simulink model "simulation_w_switch_sln3"  (Simulink 10.1)
settings: Solver=VariableStepAuto  StartTime=0.0  StopTime=tTot  MaxStep=1e-5  RelTol=1e-5
PreLoadFcn:
  | syst_init
values from neighbouring files (symbols this model uses):
  Aij = Aconn-Aii    [syst_init.m]
  AL = blkdiag(DGU.ALi)    [syst_init.m]
  atk24 = [zeros(3,1); 0.1*rand(3,1)-0.05]    [syst_init.m]
  atk34 = [zeros(3,1); 0.1*rand(3,1)-0.05]    [syst_init.m]
  B = blkdiag(DGU.B)    [syst_init.m]
  bC = blkdiag(DGU.bC)    [syst_init.m]
  bF = blkdiag(DGU.bF)    [syst_init.m]
  bH = blkdiag(DGU.bH)    [syst_init.m]
  bigCyComm = [zeros(3,3)  eye(3) zeros(3,30) ... (first row only)    [syst_init.m]
  bKhat = blkdiag(DGU.bKhat)    [syst_init.m]
  DGU = stateDyn(DGU,6)    [syst_init.m]
  F = blkdiag(DGU.Fj)    [syst_init.m]
  H = blkdiag(DGU.Hj)    [syst_init.m]
  K = blkdiag(DGU.K)    [syst_init.m]
  Khat = blkdiag(DGU.Khat)    [syst_init.m]
  L = blkdiag(DGU.Li)    [syst_init.m]
  n = 3    [syst_init.m]
  N = 6    [syst_init.m]
  nMaxMeas = .01    (= 0.01)    [syst_init.m]
  rhoMax = nMaxMeas*repmat([ones(n-1,1);0],N,1)    [syst_init.m]
  T = blkdiag(DGU.Tj)    [syst_init.m]
  Ta = 8    [syst_init.m]
  Tc = 2    [syst_init.m]
  tSampData = 1e-3    (= 0.001)    [syst_init.m]
  Vs = 60    [syst_init.m]
  wMax = nMax*repmat([ones(n-1,1);0],N,1)+nMaxMeas*repmat([zeros(n-1,1);1],N,1)    [syst_init.m]
undefined symbols (not defined in the file or in its folder): epsilon0bar, integral_Loc, rLoc_bar
libraries: powerlib x136, powerlib_meascontrol x13
(part 2 of 4)

== system simulation_w_switch_sln3/DGU5 ==
  note: Noisy Measurements
  note: State Computation
  note: Average Dynamics
  AC Current Source : powerlib/Electrical Sources/AC Current Source  Amplitude=18  Phase=90  Frequency=0  SampleTime=0  Measurements=Current
      settings: SourceProductBaseCode=PS
  Attack Detection Logic : Subsystem
  Capacitance : powerlib/Elements/Series RLC Branch  LConnTagsString=__new0  RConnTagsString=__new0  BranchType=C  Resistance=1  Inductance=1.8e-3  SetiL0=off  InitialCurrent=0  Capacitance=DGU(5).Ct  Setx0=off  InitialVoltage=48  Measurements=Branch voltage and current
  Current Measurement : powerlib/Measurements/Current Measurement  PhasorSimulation=off  OutputType=Magnitude  PSBequivalent=0
  DC Voltage Source : powerlib/Electrical Sources/DC Voltage Source  Amplitude=Vs  Measurements=Voltage
  Diode : powerlib/Power Electronics/Diode  Ron=0.001  Lon=0  Vf=0.8  IC=0  UseSnubber=0  Rs=500  Cs=250e-9  Measurements=off
  Diode1 : powerlib/Power Electronics/Diode  Ron=0.001  Lon=0  Vf=0.8  IC=0  UseSnubber=0  Rs=500  Cs=250e-9  Measurements=off
  Gain1 : Gain  Gain=[1 0 0]  Multiplication=Matrix(K*u) (u vector)
  Gain4 : Gain  Gain=[zeros(3,n*4) eye(3) zeros(3,n*1)]  Multiplication=Matrix(K*u) (u vector)
  Ground : powerlib/Elements/Ground  LConnTagsString=a
  Ground1 : powerlib/Elements/Ground  LConnTagsString=a
  IGBT : powerlib/Power Electronics/IGBT  Ron=0.001  Lon=0  Vf=1  Tf=1e-6  Tt=2e-6  IC=0  Rs=1e5  Cs=inf  Measurements=on
  IGBT1 : powerlib/Power Electronics/IGBT  Ron=0.001  Lon=0  Vf=1  Tf=1e-6  Tt=2e-6  IC=0  Rs=1e5  Cs=inf  Measurements=on
  Inductance : powerlib/Elements/Series RLC Branch  LConnTagsString=__new0  RConnTagsString=__new0  BranchType=L  Resistance=1  Inductance=DGU(5).Lt  SetiL0=off  InitialCurrent=18  Capacitance=1e-6  Setx0=off  InitialVoltage=0  Measurements=None
  Integrator : Integrator
  Luenberger  Observer : Subsystem
  Multimeter : powerlib/Measurements/Multimeter  PhasorSimulation=off  OutputType=Complex  sel=11  L=30  Gain=1  yselected={'Usrc: DGU5/DC Voltage Source'};  PSBOutputType=1  PSBequivalent=0  AxesSetting=[0,0.1,-100,100]  Display=0  SavedBlockNames=-11
  Multimeter1 : powerlib/Measurements/Multimeter  PhasorSimulation=off  OutputType=Complex  sel=18  L=30  Gain=1  yselected={'Ib: DGU5/Resistance'};  PSBOutputType=1  PSBequivalent=0  AxesSetting=[0,0.1,-100,100]  Display=0  SavedBlockNames=-11
  Multimeter2 : powerlib/Measurements/Multimeter  PhasorSimulation=off  OutputType=Complex  sel=17  L=30  Gain=1  yselected={'Ib: DGU5/Capacitance'};  PSBOutputType=1  PSBequivalent=0  AxesSetting=[0,0.1,-100,100]  Display=0  SavedBlockNames=-11
  Multimeter3 : powerlib/Measurements/Multimeter  PhasorSimulation=off  OutputType=Complex  sel=29  L=30  Gain=1  yselected={'Isrc: DGU5/AC Current Source'};  PSBOutputType=1  PSBequivalent=0  AxesSetting=[0,0.1,-100,100]  Display=0  SavedBlockNames=-11
  Multimeter5 : powerlib/Measurements/Multimeter  PhasorSimulation=off  OutputType=Complex  sel=3  L=30  Gain=1  yselected={'Ub: DGU5/Capacitance'};  PSBOutputType=1  PSBequivalent=0  AxesSetting=[0,0.1,-100,100]  Display=0  SavedBlockNames=-11
  Mux1 : Mux
  Mux4 : Mux  Inputs=3
  Primary  Voltage  Controller : Subsystem
  Product : Product  Multiplication=Matrix(*)
  Resistance : powerlib/Elements/Series RLC Branch  LConnTagsString=__new0  RConnTagsString=__new0  BranchType=R  Resistance=DGU(5).Rt  Inductance=1e-3  SetiL0=off  InitialCurrent=0  Capacitance=1e-6  Setx0=off  InitialVoltage=0  Measurements=Branch current
  Scope{,1..4,7} (6 alike) : Scope
  Secondary Consensus Layer : Subsystem
  State-Space1 : StateSpace  A=DGU(5).Aii  B=[DGU(5).M DGU(5).B [-1/DGU(5).Ct;0;0]]  C=eye(3)  D=zeros(n,4)  InitialCondition=0
  Sum2 : Sum  Inputs=|++
  Sum3 : Sum  Inputs=|+-
  Switching : Subsystem
  To Workspace : ToWorkspace  Commented=on  VariableName=x5  SaveFormat=Timeseries  SampleTime=tSampData
  To Workspace1 : ToWorkspace  Commented=on  VariableName=y5  SaveFormat=Timeseries  SampleTime=tSampData
  UIO : Subsystem
  Voltage Measurement : powerlib/Measurements/Voltage Measurement  PhasorSimulation=off  OutputType=Complex  PSBequivalent=0
  powergui1 : powerlib/powergui  Priority=1  Commented=on  SimulationMode=Continuous  SampleTime=50e-6  frequency=60  Iterations=50  frequencyindice=60  Pbase=100e6  ErrMax=1e-4  UnitsV=kV  UnitsW=MW  buscounter=0  FunctionMessages=off  echomessages=off  EnableUseOfTLC=off  CurrentSourceSwitches=off  DisableSnubberDevices=off  DisableRonSwitches=off  DisableVfSwitches=off  DisplayEquations=off  AutomaticDiscreteSolvers=off  SolverType=Tustin/Backward Euler (TBE)  Interpol=off  ExternalGateDelay=off  methode=off  Ts=100  x0status=blocks  SPID=on  SwTol=0  HookPort=off  NonlinearTolerance=1e-4  nMaxIteration=100  ContinueOnMaxIteration=off  RestoreLinks=warning  ResistiveCurrentMeasurement=off  Frange=[0:2:500]  Ylog=off  Xlog=on  ShowGrid=off  save=off  variable=ZData  structure=0  ZoomFFT=off  StartTime=0.0  cycles=1  DisplayStyle=1  fundamental=60  FreqAxis=off  MaxFrequency=1000  frequencyindicesteady=1  RmsSteady=1  display=off
  PCC5 : PMIOPort  Tag=PMCPort  Side=Left
  tag scope: Ic5=global, Il5=global, Inet5=global, It5=global, V5=global, Vs5=global, Vt5=global, x5=global, xavg5=global, y5=global
  wires:
  Multimeter/1 -> Scope/1, [Vs5]
  Multimeter2/1 -> Scope2/1, [Ic5]
  Voltage Measurement/1 -> Scope4/1, [Vt5]
  Multimeter1/1 -> Scope1/1, [It5]
  [SW_Buck_5n] -> IGBT1/1
  Multimeter3/1 -> Scope3/1, [Il5]
  [SW_Buck_5] -> IGBT/1
  Multimeter5/1 -> [V5]
  [x5] -> Sum2/2
  Sum3/1 -> Integrator/1
  Mux4/1 -> To Workspace/1, [x5]
  Sum2/1 -> To Workspace1/1, [y5]
  Integrator/1 -> Mux4/3
  Gain1/1 -> Sum3/2
  [It5] -> Mux4/2
  Gain4/1 -> Sum2/1, Scope7/1
  [y5] -> Gain1/1
  [Vref5] -> Sum3/1
  [rho] -> Gain4/1
  [V5] -> Mux4/1
  [Il5] -> Mux1/1
  Mux1/1 -> State-Space1/1
  [secondary] -> Product/2
  Current Measurement/1 -> [Inet5]
  Product/1 -> Mux1/4
  [Inet5] -> Product/1
  [Vref5] -> Mux1/2
  [Vt5d] -> Mux1/3
  State-Space1/1 -> [xavg5]
  connections:
  Ground1/LConn1 -- Voltage Measurement/LConn2
  IGBT1/RConn1 -- AC Current Source/RConn1 -- Capacitance/RConn1 -- Ground/LConn1 -- DC Voltage Source/LConn1 -- Diode1/LConn1
  Capacitance/LConn1 -- Current Measurement/LConn1 -- AC Current Source/LConn1 -- Inductance/RConn1
  IGBT/LConn1 -- Diode/RConn1 -- DC Voltage Source/RConn1
  Resistance/RConn1 -- Inductance/LConn1
  IGBT/RConn1 -- Resistance/LConn1 -- Voltage Measurement/LConn1 -- Diode1/RConn1 -- IGBT1/LConn1 -- Diode/LConn1
  PCC5/RConn1 -- Current Measurement/RConn1

== system simulation_w_switch_sln3/DGU6 ==
  note: Noisy Measurements
  note: State Computation
  note: Average Dynamics
  AC Current Source : powerlib/Electrical Sources/AC Current Source  Amplitude=16  Phase=90  Frequency=0  SampleTime=0  Measurements=Current
      settings: SourceProductBaseCode=PS
  Attack Detection Logic : Subsystem
  Capacitance : powerlib/Elements/Series RLC Branch  LConnTagsString=__new0  RConnTagsString=__new0  BranchType=C  Resistance=1  Inductance=1.8e-3  SetiL0=off  InitialCurrent=0  Capacitance=DGU(6).Ct  Setx0=off  InitialVoltage=48  Measurements=Branch voltage and current
  Current Measurement : powerlib/Measurements/Current Measurement  PhasorSimulation=off  OutputType=Magnitude  PSBequivalent=0
  DC Voltage Source : powerlib/Electrical Sources/DC Voltage Source  Amplitude=Vs  Measurements=Voltage
  Diode : powerlib/Power Electronics/Diode  Ron=0.001  Lon=0  Vf=0.8  IC=0  UseSnubber=0  Rs=500  Cs=250e-9  Measurements=off
  Diode1 : powerlib/Power Electronics/Diode  Ron=0.001  Lon=0  Vf=0.8  IC=0  UseSnubber=0  Rs=500  Cs=250e-9  Measurements=off
  Gain1 : Gain  Gain=[1 0 0]  Multiplication=Matrix(K*u) (u vector)
  Gain4 : Gain  Gain=[zeros(3,n*5) eye(3)]  Multiplication=Matrix(K*u) (u vector)
  Ground : powerlib/Elements/Ground  LConnTagsString=a
  Ground1 : powerlib/Elements/Ground  LConnTagsString=a
  IGBT : powerlib/Power Electronics/IGBT  Ron=0.001  Lon=0  Vf=1  Tf=1e-6  Tt=2e-6  IC=0  Rs=1e5  Cs=inf  Measurements=on
  IGBT1 : powerlib/Power Electronics/IGBT  Ron=0.001  Lon=0  Vf=1  Tf=1e-6  Tt=2e-6  IC=0  Rs=1e5  Cs=inf  Measurements=on
  Inductance : powerlib/Elements/Series RLC Branch  LConnTagsString=__new0  RConnTagsString=__new0  BranchType=L  Resistance=1  Inductance=DGU(6).Lt  SetiL0=off  InitialCurrent=16  Capacitance=1e-6  Setx0=off  InitialVoltage=0  Measurements=None
  Integrator : Integrator
  Luenberger  Observer1 : Subsystem
  Multimeter : powerlib/Measurements/Multimeter  PhasorSimulation=off  OutputType=Complex  sel=12  L=30  Gain=1  yselected={'Usrc: DGU6/DC Voltage Source'};  PSBOutputType=1  PSBequivalent=0  AxesSetting=[0,0.1,-100,100]  Display=0  SavedBlockNames=-11
  Multimeter1 : powerlib/Measurements/Multimeter  PhasorSimulation=off  OutputType=Complex  sel=20  L=30  Gain=1  yselected={'Ib: DGU6/Resistance'};  PSBOutputType=1  PSBequivalent=0  AxesSetting=[0,0.1,-100,100]  Display=0  SavedBlockNames=-11
  Multimeter2 : powerlib/Measurements/Multimeter  PhasorSimulation=off  OutputType=Complex  sel=19  L=30  Gain=1  yselected={'Ib: DGU6/Capacitance'};  PSBOutputType=1  PSBequivalent=0  AxesSetting=[0,0.1,-100,100]  Display=0  SavedBlockNames=-11
  Multimeter3 : powerlib/Measurements/Multimeter  PhasorSimulation=off  OutputType=Complex  sel=30  L=30  Gain=1  yselected={'Isrc: DGU6/AC Current Source'};  PSBOutputType=1  PSBequivalent=0  AxesSetting=[0,0.1,-100,100]  Display=0  SavedBlockNames=-11
  Multimeter6 : powerlib/Measurements/Multimeter  PhasorSimulation=off  OutputType=Complex  sel=4  L=30  Gain=1  yselected={'Ub: DGU6/Capacitance'};  PSBOutputType=1  PSBequivalent=0  AxesSetting=[0,0.1,-100,100]  Display=0  SavedBlockNames=-11
  Mux1 : Mux
  Mux4 : Mux  Inputs=3
  Primary  Voltage  Controller : Subsystem
  Product : Product  Multiplication=Matrix(*)
  Resistance : powerlib/Elements/Series RLC Branch  LConnTagsString=__new0  RConnTagsString=__new0  BranchType=R  Resistance=DGU(6).Rt  Inductance=1e-3  SetiL0=off  InitialCurrent=0  Capacitance=1e-6  Setx0=off  InitialVoltage=0  Measurements=Branch current
  Scope{,1..4,7} (6 alike) : Scope
  Secondary Consensus Layer : Subsystem
  State-Space1 : StateSpace  A=DGU(6).Aii  B=[DGU(6).M DGU(6).B [-1/DGU(6).Ct;0;0]]  C=eye(3)  D=zeros(n,4)  InitialCondition=0
  Sum2 : Sum  Inputs=|++
  Sum3 : Sum  Inputs=|+-
  Switching : Subsystem
  To Workspace : ToWorkspace  Commented=on  VariableName=x6  SaveFormat=Timeseries  SampleTime=tSampData
  To Workspace1 : ToWorkspace  Commented=on  VariableName=y6  SaveFormat=Timeseries  SampleTime=tSampData
  UIO1 : Subsystem
  Voltage Measurement : powerlib/Measurements/Voltage Measurement  PhasorSimulation=off  OutputType=Complex  PSBequivalent=0
  powergui1 : powerlib/powergui  Priority=1  Commented=on  SimulationMode=Continuous  SampleTime=50e-6  frequency=60  Iterations=50  frequencyindice=60  Pbase=100e6  ErrMax=1e-4  UnitsV=kV  UnitsW=MW  buscounter=0  FunctionMessages=off  echomessages=off  EnableUseOfTLC=off  CurrentSourceSwitches=off  DisableSnubberDevices=off  DisableRonSwitches=off  DisableVfSwitches=off  DisplayEquations=off  AutomaticDiscreteSolvers=off  SolverType=Tustin/Backward Euler (TBE)  Interpol=off  ExternalGateDelay=off  methode=off  Ts=100  x0status=blocks  SPID=on  SwTol=0  HookPort=off  NonlinearTolerance=1e-4  nMaxIteration=100  ContinueOnMaxIteration=off  RestoreLinks=warning  ResistiveCurrentMeasurement=off  Frange=[0:2:500]  Ylog=off  Xlog=on  ShowGrid=off  save=off  variable=ZData  structure=0  ZoomFFT=off  StartTime=0.0  cycles=1  DisplayStyle=1  fundamental=60  FreqAxis=off  MaxFrequency=1000  frequencyindicesteady=1  RmsSteady=1  display=off
  PCC6 : PMIOPort  Tag=PMCPort  Side=Right
  tag scope: Ic6=global, Il6=global, Inet6=global, It6=global, V6=global, Vs6=global, Vt6=global, x6=global, xavg6=global, y6=global
  wires:
  Multimeter/1 -> Scope/1, [Vs6]
  Multimeter2/1 -> Scope2/1, [Ic6]
  Voltage Measurement/1 -> Scope4/1, [Vt6]
  Multimeter1/1 -> Scope1/1, [It6]
  [SW_Buck_6n] -> IGBT1/1
  Multimeter3/1 -> Scope3/1, [Il6]
  [SW_Buck_6] -> IGBT/1
  Multimeter6/1 -> [V6]
  [x6] -> Sum2/2
  Sum3/1 -> Integrator/1
  Mux4/1 -> To Workspace/1, [x6]
  Sum2/1 -> To Workspace1/1, [y6]
  Integrator/1 -> Mux4/3
  Gain1/1 -> Sum3/2
  [It6] -> Mux4/2
  Gain4/1 -> Sum2/1, Scope7/1
  [y6] -> Gain1/1
  [Vref6] -> Sum3/1
  [rho] -> Gain4/1
  [V6] -> Mux4/1
  [Il6] -> Mux1/1
  Mux1/1 -> State-Space1/1
  [secondary] -> Product/2
  Current Measurement/1 -> [Inet6]
  Product/1 -> Mux1/4
  [Inet6] -> Product/1
  [Vref6] -> Mux1/2
  [Vt6d] -> Mux1/3
  State-Space1/1 -> [xavg6]
  connections:
  Ground1/LConn1 -- Voltage Measurement/LConn2
  IGBT1/RConn1 -- AC Current Source/RConn1 -- Capacitance/RConn1 -- Ground/LConn1 -- DC Voltage Source/LConn1 -- Diode1/LConn1
  Capacitance/LConn1 -- Current Measurement/LConn1 -- AC Current Source/LConn1 -- Inductance/RConn1
  IGBT/LConn1 -- Diode/RConn1 -- DC Voltage Source/RConn1
  Resistance/RConn1 -- Inductance/LConn1
  IGBT/RConn1 -- Resistance/LConn1 -- Voltage Measurement/LConn1 -- Diode1/RConn1 -- IGBT1/LConn1 -- Diode/LConn1
  PCC6/RConn1 -- Current Measurement/RConn1

== system simulation_w_switch_sln3/Luenberger Thresholds ==
  Abs : Abs
  Clock : Clock  Commented=on
  Constant : Constant  Commented=on  Value=zeros(n,1)
  From Workspace1 : FromWorkspace  VariableName=rLoc_bar_ts
  From2 : From  Commented=on  GotoTag=secondary  TagVisibility=global
  Integrator : Integrator  Commented=on  ExternalReset=rising
  Interpreted MATLAB Function1 : MATLABFcn  Commented=on  MATLABFcn=abs(expm(AL*(u(end)-Tc)))*epsilon0bar + rhoMax + abs(expm(AL*u(end)))*(abs(Aij)*rhoMax + wMax + abs(L)*rhoMax)
  MATLAB Function : MATLAB Function  Commented=on  TreatAsAtomicUnit=on
  Mux : Mux  Commented=on  Inputs=2
  Product : Product  Multiplication=Matrix(*)
  Product1 : Product  Commented=on  Multiplication=Matrix(*)
  Scope : Scope  Commented=on  NumInputPorts=2
  Sum6 : Sum  Inputs=+|-
  Switch : Switch  Commented=on  Criteria=u2 > Threshold  Threshold=0.1
  exponential : MATLABFcn  Commented=on  MATLABFcn=abs(expm(-AL*u))
  integral_Loc : MATLABFcn  Commented=on  MATLABFcn=integral_Loc(u,AL)
  rLoc_bar : MATLABFcn  Commented=on  MATLABFcn=rLoc_bar(u,Tc,AL,Aij,L,rhoMax,wMax,epsilon0bar)
  tag scope: rLoc1=global, rLoc_bar=global
  wires:
  Product1/1 -> ?
  Clock/1 -> integral_Loc/1, Mux/2
  Abs/1 -> Product/1
  Sum6/1 -> Abs/1
  [xhat1] -> Sum6/2
  [x1] -> Sum6/1
  Constant/1 -> Switch/3
  Product/1 -> [rLoc1]
  [secondary] -> Product/2
  integral_Loc/1 -> Integrator/1
  Integrator/1 -> Mux/1, Scope/1
  From2/1 -> Integrator/2, Product1/2
  rLoc_bar/1 -> Product1/1
  Mux/1 -> Scope/2, rLoc_bar/1
  From Workspace1/1 -> [rLoc_bar]

== system simulation_w_switch_sln3/UIO Thresholds ==
  Abs : Abs
  From Workspace1 : FromWorkspace  VariableName=r_bar_ts
  Gain2 : Gain  Gain=[eye(3) zeros(3,15)]  Multiplication=Matrix(K*u) (u vector)
  Product : Product  Multiplication=Matrix(*)
  Sum6 : Sum  Inputs=+|-
  tag scope: r12=global, r_bar=global
  wires:
  Abs/1 -> Product/1
  Sum6/1 -> Abs/1
  Gain2/1 -> Sum6/2
  [x1] -> Sum6/1
  Product/1 -> [r12]
  [secondary] -> Product/2
  From Workspace1/1 -> [r_bar]
  [y_j2_hat] -> Gain2/1

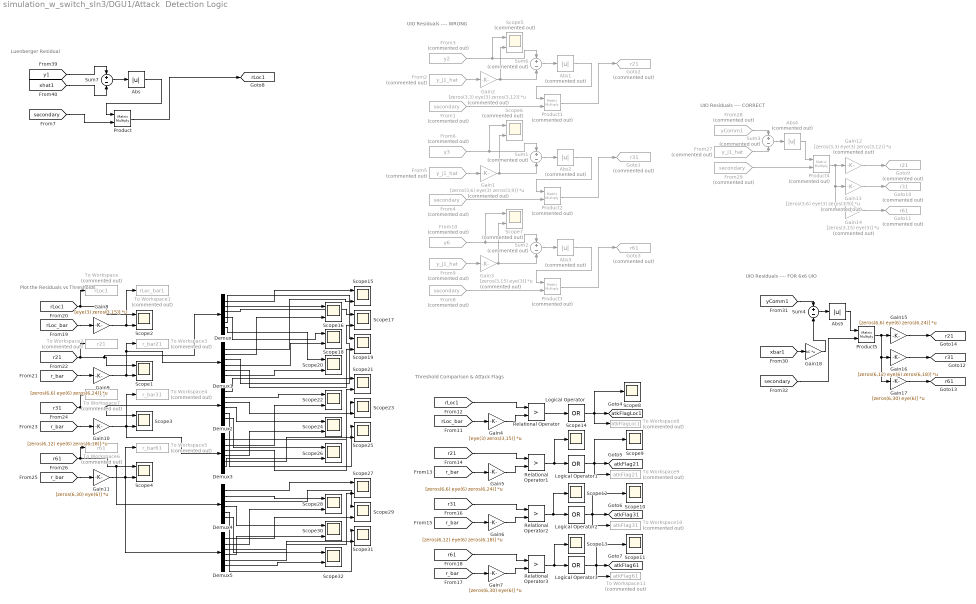
== system simulation_w_switch_sln3/DGU1/Attack  Detection Logic ==
  note: UIO Residuals ---- CORRECT
  note: Threshold Comparison & Attack Flags
  note: UIO Residuals ---- WRONG
  note: Luenberger Residual
  note: Plot the Residuals vs Thresholds
  note: UIO Residuals ---- FOR 6x6 UIO
  Abs : Abs
  Abs{1..4} (4 alike) : Abs  Commented=on
  Abs5 : Abs  ZeroCross=off
  Demux{,1..5} (6 alike) : Demux  Outputs=6
  From{1,4,8,29} (4 alike) : From  Commented=on  GotoTag=secondary  TagVisibility=global
  From10 : From  Commented=on  GotoTag=y6  TagVisibility=global
  From{2,5,9,27} (4 alike) : From  Commented=on  GotoTag=y_j1_hat  TagVisibility=global
  From28 : From  Commented=on  GotoTag=yComm1  TagVisibility=global
  From3 : From  Commented=on  GotoTag=y2  TagVisibility=global
  From6 : From  Commented=on  GotoTag=y3  TagVisibility=global
  Gain1 : Gain  Commented=on  Gain=[zeros(3,6) eye(3) zeros(3,9)]  Multiplication=Matrix(K*u) (u vector)
  Gain10 : Gain  Gain=[zeros(6,12) eye(6) zeros(6,18)]  Multiplication=Matrix(K*u) (u vector)
  Gain11 : Gain  Gain=[zeros(6,30) eye(6)]  Multiplication=Matrix(K*u) (u vector)
  Gain12 : Gain  Commented=on  Gain=[zeros(3,3) eye(3) zeros(3,12)]  Multiplication=Matrix(K*u) (u vector)
  Gain13 : Gain  Commented=on  Gain=[zeros(3,6) eye(3) zeros(3,9)]  Multiplication=Matrix(K*u) (u vector)
  Gain14 : Gain  Commented=on  Gain=[zeros(3,15) eye(3)]  Multiplication=Matrix(K*u) (u vector)
  Gain15 : Gain  Gain=[zeros(6,6) eye(6) zeros(6,24)]  Multiplication=Matrix(K*u) (u vector)
  Gain16 : Gain  Gain=[zeros(6,12) eye(6) zeros(6,18)]  Multiplication=Matrix(K*u) (u vector)
  Gain17 : Gain  Gain=[zeros(6,30) eye(6)]  Multiplication=Matrix(K*u) (u vector)
  Gain18 : Gain  Gain=bC  Multiplication=Matrix(K*u) (u vector)
  Gain2 : Gain  Commented=on  Gain=[zeros(3,3) eye(3) zeros(3,12)]  Multiplication=Matrix(K*u) (u vector)
  Gain3 : Gain  Commented=on  Gain=[zeros(3,15) eye(3)]  Multiplication=Matrix(K*u) (u vector)
  Gain4 : Gain  Gain=[eye(3) zeros(3,15)]  Multiplication=Matrix(K*u) (u vector)
  Gain5 : Gain  Gain=[zeros(6,6) eye(6) zeros(6,24)]  Multiplication=Matrix(K*u) (u vector)
  Gain6 : Gain  Gain=[zeros(6,12) eye(6) zeros(6,18)]  Multiplication=Matrix(K*u) (u vector)
  Gain7 : Gain  Gain=[zeros(6,30) eye(6)]  Multiplication=Matrix(K*u) (u vector)
  Gain8 : Gain  Gain=[eye(3) zeros(3,15)]  Multiplication=Matrix(K*u) (u vector)
  Gain9 : Gain  Gain=[zeros(6,6) eye(6) zeros(6,24)]  Multiplication=Matrix(K*u) (u vector)
  Goto1 : Goto  Commented=on  GotoTag=r31  TagVisibility=global
  Goto10 : Goto  Commented=on  GotoTag=r31  TagVisibility=global
  Goto11 : Goto  Commented=on  GotoTag=r61  TagVisibility=global
  Goto2 : Goto  Commented=on  GotoTag=r21  TagVisibility=global
  Goto3 : Goto  Commented=on  GotoTag=r61  TagVisibility=global
  Goto9 : Goto  Commented=on  GotoTag=r21  TagVisibility=global
  Logical Operator{,1..3} (4 alike) : Logic  Operator=OR  Inputs=1  AllPortsSameDT=off  OutDataTypeStr=boolean
  Product : Product  Multiplication=Matrix(*)
  Product{1..4} (4 alike) : Product  Commented=on  Multiplication=Matrix(*)
  Product5 : Product  Multiplication=Matrix(*)
  Relational Operator{,1..3} (4 alike) : RelationalOperator  Operator=>  OutDataTypeStr=boolean  RndMeth=Simplest
  Scope{1..4,15..32} (22 alike) : Scope  NumInputPorts=2
  Scope{8..14} (7 alike) : Scope
  Scope5 : Scope  Commented=on  NumInputPorts=2
  Scope6 : Scope  Commented=on  NumInputPorts=2
  Scope7 : Scope  Commented=on  NumInputPorts=2
  Sum{1..3,6} (4 alike) : Sum  Commented=on  Inputs=+|-
  Sum4 : Sum  Inputs=+|-
  Sum7 : Sum  Inputs=+|-
  To Workspace : ToWorkspace  Commented=on  VariableName=rLoc1  SaveFormat=Timeseries  SampleTime=tSampData
  To Workspace1 : ToWorkspace  Commented=on  VariableName=rLoc_bar1  SaveFormat=Timeseries  SampleTime=tSampData
  To Workspace10 : ToWorkspace  Commented=on  VariableName=atkFlag31  SaveFormat=Timeseries  SampleTime=tSampData
  To Workspace11 : ToWorkspace  Commented=on  VariableName=atkFlag61  SaveFormat=Timeseries  SampleTime=tSampData
  To Workspace2 : ToWorkspace  Commented=on  VariableName=r21  SaveFormat=Timeseries  SampleTime=tSampData
  To Workspace3 : ToWorkspace  Commented=on  VariableName=r_bar21  SaveFormat=Timeseries  SampleTime=tSampData
  To Workspace4 : ToWorkspace  Commented=on  VariableName=r_bar31  SaveFormat=Timeseries  SampleTime=tSampData
  To Workspace5 : ToWorkspace  Commented=on  VariableName=r_bar61  SaveFormat=Timeseries  SampleTime=tSampData
  To Workspace6 : ToWorkspace  Commented=on  VariableName=r61  SaveFormat=Timeseries  SampleTime=tSampData
  To Workspace7 : ToWorkspace  Commented=on  VariableName=r31  SaveFormat=Timeseries  SampleTime=tSampData
  To Workspace8 : ToWorkspace  Commented=on  VariableName=atkFlagLoc1  SaveFormat=Timeseries  SampleTime=tSampData
  To Workspace9 : ToWorkspace  Commented=on  VariableName=atkFlag21  SaveFormat=Timeseries  SampleTime=tSampData
  tag scope: atkFlag21=global, atkFlag31=global, atkFlag61=global, atkFlagLoc1=global, r21=global, r31=global, r61=global, rLoc1=global
  wires:
  Sum7/1 -> Abs/1
  [y1] -> Sum7/1
  Product/1 -> [rLoc1]
  Abs/1 -> Product/1
  [secondary] -> Product/2
  [xhat1] -> Sum7/2
  Gain2/1 -> Scope5/2, Sum6/2
  From2/1 -> Gain2/1
  Product1/1 -> Goto2/1
  Sum6/1 -> Abs1/1
  From1/1 -> Product1/2
  Abs1/1 -> Product1/1
  From3/1 -> Scope5/1, Sum6/1
  From6/1 -> Scope6/1, Sum1/1
  Abs2/1 -> Product2/1
  Gain1/1 -> Sum1/2, Scope6/2
  Sum1/1 -> Abs2/1
  From4/1 -> Product2/2
  Product2/1 -> Goto1/1
  From5/1 -> Gain1/1
  From10/1 -> Scope7/1, Sum2/1
  Abs3/1 -> Product3/1
  Gain3/1 -> Scope7/2, Sum2/2
  Sum2/1 -> Abs3/1
  From8/1 -> Product3/2
  Product3/1 -> Goto3/1
  From9/1 -> Gain3/1
  [rLoc_bar] -> Gain4/1
  Gain4/1 -> Relational Operator/2
  [rLoc1] -> Relational Operator/1
  Relational Operator/1 -> Logical Operator/1
  Relational Operator1/1 -> Scope14/1, Logical Operator1/1
  Gain5/1 -> Relational Operator1/2
  [r21] -> Relational Operator1/1
  [r_bar] -> Gain5/1
  Logical Operator1/1 -> To Workspace9/1, Scope9/1, [atkFlag21]
  [r_bar] -> Gain6/1
  Logical Operator2/1 -> To Workspace10/1, Scope10/1, [atkFlag31]
  [r31] -> Relational Operator2/1
  Gain6/1 -> Relational Operator2/2
  Relational Operator2/1 -> Scope12/1, Logical Operator2/1
  [r_bar] -> Gain7/1
  Logical Operator3/1 -> To Workspace11/1, Scope11/1, [atkFlag61]
  [r61] -> Relational Operator3/1
  Gain7/1 -> Relational Operator3/2
  Relational Operator3/1 -> Scope13/1, Logical Operator3/1
  Logical Operator/1 -> To Workspace8/1, Scope8/1, [atkFlagLoc1]
  [rLoc_bar] -> Gain8/1
  [r_bar] -> Gain11/1
  [rLoc1] -> Scope2/1, To Workspace/1
  Gain11/1 -> To Workspace5/1, Demux5/1, Scope4/2
  [r_bar] -> Gain9/1
  Gain9/1 -> To Workspace3/1, Demux1/1, Scope1/2
  [r21] -> To Workspace2/1, Demux/1, Scope1/1
  Gain8/1 -> To Workspace1/1, Scope2/2
  Gain10/1 -> To Workspace4/1, Demux3/1, Scope3/2
  [r31] -> To Workspace7/1, Scope3/1, Demux2/1
  [r_bar] -> Gain10/1
  [r61] -> To Workspace6/1, Demux4/1, Scope4/1
  From28/1 -> Sum3/1
  From27/1 -> Sum3/2
  Sum3/1 -> Abs4/1
  Abs4/1 -> Product4/1
  From29/1 -> Product4/2
  Product4/1 -> Gain14/1, Gain13/1, Gain12/1
  Gain12/1 -> Goto9/1
  Gain13/1 -> Goto10/1
  Gain14/1 -> Goto11/1
  Gain17/1 -> [r61]
  Gain16/1 -> [r31]
  Gain15/1 -> [r21]
  Product5/1 -> Gain15/1, Gain16/1, Gain17/1
  [secondary] -> Product5/2
  Abs5/1 -> Product5/1
  Sum4/1 -> Abs5/1
  [yComm1] -> Sum4/1
  [xbar1] -> Gain18/1
  Gain18/1 -> Sum4/2
  Demux/1 -> Scope15/1
  Demux1/1 -> Scope15/2
  Demux/2 -> Scope16/1
  Demux1/2 -> Scope16/2
  Demux/3 -> Scope17/1
  Demux1/3 -> Scope17/2
  Demux/4 -> Scope18/1
  Demux1/4 -> Scope18/2
  Demux/5 -> Scope19/1
  Demux1/5 -> Scope19/2
  Demux/6 -> Scope20/1
  Demux1/6 -> Scope20/2
  Demux2/1 -> Scope21/1
  Demux3/1 -> Scope21/2
  Demux2/2 -> Scope22/1
  Demux3/2 -> Scope22/2
  Demux2/3 -> Scope23/1
  Demux3/3 -> Scope23/2
  Demux2/4 -> Scope24/1
  Demux3/4 -> Scope24/2
  Demux2/5 -> Scope25/1
  Demux3/5 -> Scope25/2
  Demux2/6 -> Scope26/1
  Demux3/6 -> Scope26/2
  Demux4/1 -> Scope27/1
  Demux5/1 -> Scope27/2
  Demux4/2 -> Scope28/1
  Demux5/2 -> Scope28/2
  Demux4/3 -> Scope29/1
  Demux5/3 -> Scope29/2
  Demux4/4 -> Scope30/1
  Demux5/4 -> Scope30/2
  Demux4/5 -> Scope31/1
  Demux5/5 -> Scope31/2
  Demux4/6 -> Scope32/1
  Demux5/6 -> Scope32/2

== system simulation_w_switch_sln3/DGU1/Luenberger  Observer ==
  Enabled  Luenberger : Subsystem
      settings: MinAlgLoopOccurrences=on
  Gain1 : Gain  Gain=bigCyComm  Multiplication=Matrix(K*u) (u vector)
  Gain17 : Gain  Gain=[DGU(1).B , DGU(1).Li , DGU(1).M , Aij(1:n,:)]  Multiplication=Matrix(K*u) (u vector)
  Gain18 : Gain  Gain=DGU(1).A-DGU(1).Li*DGU(1).C  Multiplication=Matrix(K*u) (u vector)
  Integrator4 : Integrator  ExternalReset=rising  InitialConditionSource=external  InitialCondition=[0;0;0]
  Mux : Mux  Inputs=5
  Product4 : Product  Multiplication=Matrix(*)
  State-Space : StateSpace  A=DGU(1).A-DGU(1).Li*DGU(1).C  B=[DGU(1).B , DGU(1).Li , DGU(1).M , Aij(1:n,:)]  C=eye(3)  D=zeros(n,n+3+n*N)  InitialCondition=zeros(n,1)
  Sum10 : Sum  Inputs=++|
  tag scope: xhat1=global
  wires:
  [secondary] -> Enabled  Luenberger/Enable
  Product4/1 -> [xhat1]
  [Il1] -> Mux/3
  [y1] -> Integrator4/3, Mux/2
  [Vref1] -> Mux/4
  Gain17/1 -> Sum10/2
  Gain18/1 -> Sum10/1
  [secondary] -> Integrator4/2, Product4/2
  Mux/1 -> Gain17/1
  Sum10/1 -> Integrator4/1
  Integrator4/1 -> Product4/1, Gain18/1
  [Vt1] -> Mux/1
  [yComm1] -> Gain1/1
  Gain1/1 -> Mux/5

== system simulation_w_switch_sln3/DGU1/Primary  Voltage  Controller ==
  Gain1 : Gain  Gain=DGU(1).K  Multiplication=Matrix(K*u) (u vector)
  tag scope: Vt1d=global
  wires:
  Gain1/1 -> [Vt1d]
  [y1] -> Gain1/1

== system simulation_w_switch_sln3/DGU1/Secondary  Consensus  Layer ==
  note: deltaV1
  Gain : Gain  Gain=repmat([0 0 0 0 1 0],1,6)  Multiplication=Matrix(K*u) (u vector)
  Gain12 : Gain  Gain=DGU(1).kI
  Gain6 : Gain  Gain=length(DGU(1).Ni)
  Integrator : Integrator  ExternalReset=rising
  Sum6 : Sum  Inputs=|+-
  Sum7 : Sum  Inputs=|++
  Switch : Switch  Criteria=u2 > Threshold  Threshold=0.1
  tag scope: Vref1=global
  wires:
  [secondary] -> Integrator/2, Switch/2
  [yComm1] -> Gain/1
  Gain/1 -> Sum6/1
  Sum7/1 -> Switch/1
  Integrator/1 -> Sum7/1
  Switch/1 -> [Vref1]
  [Vref] -> Switch/3, Sum7/2
  [It1] -> Gain6/1
  Gain6/1 -> Sum6/2
  Sum6/1 -> Gain12/1
  Gain12/1 -> Integrator/1

== system simulation_w_switch_sln3/DGU1/Switching ==
  Divide : Product  Inputs=*/
  Logical Operator : Logic  Operator=NOT  AllPortsSameDT=off  OutDataTypeStr=boolean
  PWM Generator (DC-DC) : powerlib_meascontrol/Pulse & Signal Generators/PWM Generator (DC-DC)  Fsw=10000  Ts=0
  tag scope: SW_Buck_1=global, SW_Buck_1n=global, SW_Duty_1=global
  wires:
  [Vs1] -> Divide/2
  Logical Operator/1 -> [SW_Buck_1n]
  PWM Generator (DC-DC)/1 -> Logical Operator/1, [SW_Buck_1]
  Divide/1 -> [SW_Duty_1], PWM Generator (DC-DC)/1
  [Vt1d] -> Divide/1

== system simulation_w_switch_sln3/DGU1/UIO ==
  note: 6x6 UIO for the states of DGUs with average dynamics
  note: UIO for the states of DGU 1 with Switched Inputs - Used for debugging
  note: Single UIO for all neighbors of DGU 1 with Switched Inputs
  note: Calculated Switching Inputs
  Constant : Constant  Commented=on  Value=0.8132
  Constant1 : Constant  Commented=on  Value=Vs
  Constant2 : Constant  Commented=on  Value=0.8132
  Divide : Product  Commented=on  Inputs=*/  Multiplication=Matrix(*)
  Enabled  UIO : Subsystem  Commented=on
      settings: MinAlgLoopOccurrences=on
  From1 : From  Commented=on  GotoTag=y1C
  From12 : From  Commented=on  GotoTag=SW_Buck_1  TagVisibility=global
  From13 : From  Commented=on  GotoTag=y1  TagVisibility=global
  From15 : From  Commented=on  GotoTag=xavg1  TagVisibility=global
  From2 : From  Commented=on  GotoTag=secondary  TagVisibility=global
  From3 : From  Commented=on  GotoTag=secondary  TagVisibility=global
  From4 : From  Commented=on  GotoTag=Vt1  TagVisibility=global
  From5 : From  Commented=on  GotoTag=yComm1  TagVisibility=global
  From6 : From  Commented=on  GotoTag=yComm1  TagVisibility=global
  From7 : From  Commented=on  GotoTag=yComm1  TagVisibility=global
  From8 : From  Commented=on  GotoTag=SW_yComm1  TagVisibility=global
  From9 : From  Commented=on  GotoTag=secondary  TagVisibility=global
  Gain : Gain  Commented=on  Gain=[DGU(1).Khat DGU(1).Tj*DGU(1).B]  Multiplication=Matrix(K*u) (u vector)
  Gain1 : Gain  Commented=on  Gain=DGU(1).Fj  Multiplication=Matrix(K*u) (u vector)
  Gain14 : Gain  Commented=on  Gain=59.7999  Multiplication=Matrix(K*u) (u vector)
  Gain15 : Gain  Gain=bH  Multiplication=Matrix(K*u) (u vector)
  Gain16 : Gain  Gain=inv(bC)-bH  Multiplication=Matrix(K*u) (u vector)
  Gain17 : Gain  Gain=bKhat  Multiplication=Matrix(K*u) (u vector)
  Gain18 : Gain  Gain=bF  Multiplication=Matrix(K*u) (u vector)
  Gain2 : Gain  Commented=on  Gain=DGU(1).Hj  Multiplication=Matrix(K*u) (u vector)
  Gain3 : Gain  Commented=on  Gain=DGU(1).Tj  Multiplication=Matrix(K*u) (u vector)
  Gain4 : Gain  Commented=on  Gain=K  Multiplication=Matrix(K*u) (u vector)
  Gain5 : Gain  Commented=on  Gain=[Khat T*B]  Multiplication=Matrix(K*u) (u vector)
  Gain6 : Gain  Commented=on  Gain=F  Multiplication=Matrix(K*u) (u vector)
  Gain7 : Gain  Commented=on  Gain=59.7999
  Gain8 : Gain  Commented=on  Gain=H  Multiplication=Matrix(K*u) (u vector)
  Gain9 : Gain  Commented=on  Gain=T  Multiplication=Matrix(K*u) (u vector)
  Goto : Goto  Commented=on  GotoTag=SW_yComm1  TagVisibility=global
  Goto1 : Goto  Commented=on  GotoTag=y_j1_hat  TagVisibility=global
  Goto2 : Goto  Commented=on  GotoTag=y_j1_hatt  TagVisibility=global
  Goto3 : Goto  Commented=on  GotoTag=y_j1_hat  TagVisibility=global
  Goto4 : Goto  Commented=on  GotoTag=Duty_yComm1  TagVisibility=global
  Integrator : Integrator  Commented=on  ExternalReset=rising  InitialConditionSource=external
  Integrator1 : Integrator  Commented=on  ExternalReset=rising  InitialConditionSource=external
  Integrator4 : Integrator  ExternalReset=rising  InitialConditionSource=external  InitialCondition=[0;0;0]
  Mux1 : Mux  Commented=on  Inputs=2
  Mux2 : Mux  Commented=on  Inputs=2
  Mux3 : Mux  Commented=on  Inputs=2
  PWM Generator (DC-DC) : powerlib_meascontrol/Pulse & Signal Generators/PWM Generator (DC-DC)  Commented=on  Fsw=10000  Ts=0
  Product : Product  Commented=on  Multiplication=Matrix(*)
  Product1 : Product  Commented=on  Multiplication=Matrix(*)
  Product4 : Product  Multiplication=Matrix(*)
  Sum{,1..3} (4 alike) : Sum  Commented=on  Inputs=++|
  Sum10 : Sum  Inputs=++|
  Sum11 : Sum  Inputs=++|
  Sum4 : Sum  Commented=on  Inputs=|-+
  Sum9 : Sum  Commented=on  Inputs=|-+
  tag scope: xbar1=global
  wires:
  Enabled  UIO/1(y_ji_hat) -> Goto1/1
  From2/1 -> Enabled  UIO/Enable
  From6/1 -> Enabled  UIO/1(u)
  From15/1 -> Mux2/1
  Integrator4/1 -> Sum11/2, Gain18/1
  Gain17/1 -> Sum10/2
  Product4/1 -> [xbar1]
  Gain18/1 -> Sum10/1
  [secondary] -> Integrator4/2, Product4/2
  Sum10/1 -> Integrator4/1
  Gain15/1 -> Sum11/1
  [yComm1] -> Gain16/1, Gain15/1, Gain17/1
  Sum11/1 -> Product4/1
  From13/1 -> Mux2/2
  Constant/1 -> Sum9/1
  Gain2/1 -> Sum1/1
  Sum/1 -> Integrator/1
  Gain14/1 -> Sum9/2
  From1/1 -> Gain2/1, Gain3/1, Mux1/1
  Gain3/1 -> Integrator/3
  Mux1/1 -> Gain/1
  From12/1 -> Gain14/1
  From3/1 -> Integrator/2, Product/2
  Integrator/1 -> Sum1/2, Gain1/1
  Gain1/1 -> Sum/1
  Sum1/1 -> Product/1
  Gain/1 -> Sum/2
  Sum9/1 -> Mux1/2
  Product/1 -> Goto2/1
  PWM Generator (DC-DC)/1 -> Goto/1
  Divide/1 -> Goto4/1, PWM Generator (DC-DC)/1
  Constant1/1 -> Divide/2
  Gain4/1 -> Divide/1
  From7/1 -> Gain4/1
  Constant2/1 -> Sum4/1
  From5/1 -> Gain8/1, Gain9/1, Mux3/1
  Sum3/1 -> Product1/1
  Gain5/1 -> Sum2/2
  Gain7/1 -> Sum4/2
  From8/1 -> Gain7/1
  Mux3/1 -> Gain5/1
  Gain8/1 -> Sum3/1
  Gain9/1 -> Integrator1/3
  From9/1 -> Integrator1/2, Product1/2
  Sum2/1 -> Integrator1/1
  Sum4/1 -> Mux3/2
  Integrator1/1 -> Sum3/2, Gain6/1
  Gain6/1 -> Sum2/1
  Product1/1 -> Goto3/1
  Gain16/1 -> Integrator4/3

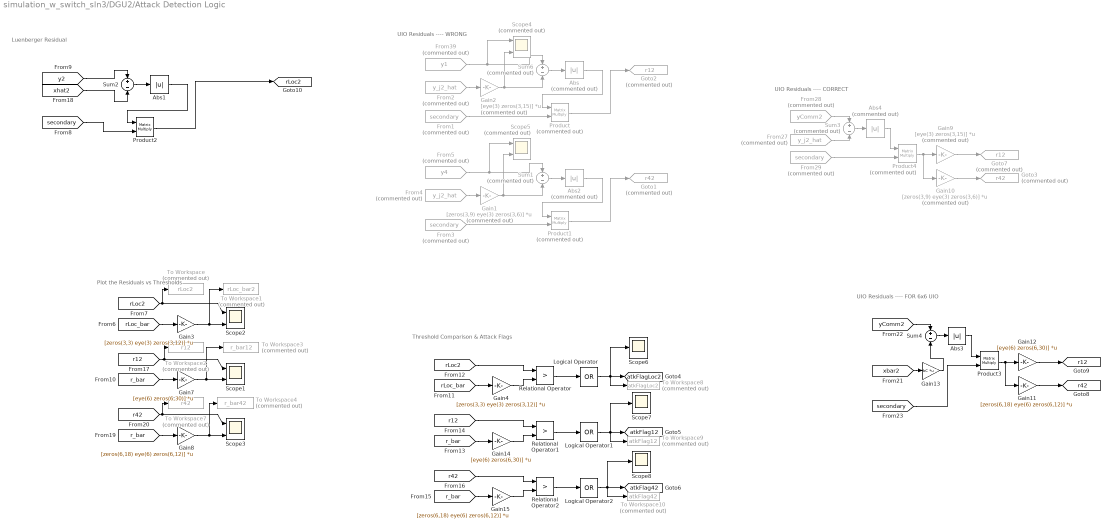
== system simulation_w_switch_sln3/DGU2/Attack Detection Logic ==
  note: UIO Residuals ---- WRONG
  note: Luenberger Residual
  note: Threshold Comparison & Attack Flags
  note: Plot the Residuals vs Thresholds
  note: UIO Residuals ---- CORRECT
  note: UIO Residuals ---- FOR 6x6 UIO
  Abs : Abs  Commented=on
  Abs1 : Abs
  Abs2 : Abs  Commented=on
  Abs3 : Abs  ZeroCross=off
  Abs4 : Abs  Commented=on
  From1 : From  Commented=on  GotoTag=secondary  TagVisibility=global
  From2 : From  Commented=on  GotoTag=y_j2_hat  TagVisibility=global
  From27 : From  Commented=on  GotoTag=y_j2_hat  TagVisibility=global
  From28 : From  Commented=on  GotoTag=yComm2  TagVisibility=global
  From29 : From  Commented=on  GotoTag=secondary  TagVisibility=global
  From3 : From  Commented=on  GotoTag=secondary  TagVisibility=global
  From39 : From  Commented=on  GotoTag=y1  TagVisibility=global
  From4 : From  Commented=on  GotoTag=y_j2_hat  TagVisibility=global
  From5 : From  Commented=on  GotoTag=y4  TagVisibility=global
  Gain1 : Gain  Commented=on  Gain=[zeros(3,9) eye(3) zeros(3,6)]  Multiplication=Matrix(K*u) (u vector)
  Gain10 : Gain  Commented=on  Gain=[zeros(3,9) eye(3) zeros(3,6)]  Multiplication=Matrix(K*u) (u vector)
  Gain11 : Gain  Gain=[zeros(6,18) eye(6) zeros(6,12)]  Multiplication=Matrix(K*u) (u vector)
  Gain12 : Gain  Gain=[eye(6) zeros(6,30)]  Multiplication=Matrix(K*u) (u vector)
  Gain13 : Gain  Gain=bC  Multiplication=Matrix(K*u) (u vector)
  Gain14 : Gain  Gain=[eye(6) zeros(6,30)]  Multiplication=Matrix(K*u) (u vector)
  Gain15 : Gain  Gain=[zeros(6,18) eye(6) zeros(6,12)]  Multiplication=Matrix(K*u) (u vector)
  Gain2 : Gain  Commented=on  Gain=[eye(3) zeros(3,15)]  Multiplication=Matrix(K*u) (u vector)
  Gain3 : Gain  Gain=[zeros(3,3) eye(3) zeros(3,12)]  Multiplication=Matrix(K*u) (u vector)
  Gain4 : Gain  Gain=[zeros(3,3) eye(3) zeros(3,12)]  Multiplication=Matrix(K*u) (u vector)
  Gain7 : Gain  Gain=[eye(6) zeros(6,30)]  Multiplication=Matrix(K*u) (u vector)
  Gain8 : Gain  Gain=[zeros(6,18) eye(6) zeros(6,12)]  Multiplication=Matrix(K*u) (u vector)
  Gain9 : Gain  Commented=on  Gain=[eye(3) zeros(3,15)]  Multiplication=Matrix(K*u) (u vector)
  Goto1 : Goto  Commented=on  GotoTag=r42  TagVisibility=global
  Goto2 : Goto  Commented=on  GotoTag=r12  TagVisibility=global
  Goto3 : Goto  Commented=on  GotoTag=r42  TagVisibility=global
  Goto7 : Goto  Commented=on  GotoTag=r12  TagVisibility=global
  Logical Operator : Logic  Operator=OR  Inputs=1  AllPortsSameDT=off  OutDataTypeStr=boolean
  Logical Operator1 : Logic  Operator=OR  Inputs=1  AllPortsSameDT=off  OutDataTypeStr=boolean
  Logical Operator2 : Logic  Operator=OR  Inputs=1  AllPortsSameDT=off  OutDataTypeStr=boolean
  Product : Product  Commented=on  Multiplication=Matrix(*)
  Product1 : Product  Commented=on  Multiplication=Matrix(*)
  Product2 : Product  Multiplication=Matrix(*)
  Product3 : Product  Multiplication=Matrix(*)
  Product4 : Product  Commented=on  Multiplication=Matrix(*)
  Relational Operator : RelationalOperator  Operator=>  OutDataTypeStr=boolean  RndMeth=Simplest
  Relational Operator1 : RelationalOperator  Operator=>  OutDataTypeStr=boolean  RndMeth=Simplest
  Relational Operator2 : RelationalOperator  Operator=>  OutDataTypeStr=boolean  RndMeth=Simplest
  Scope1 : Scope  NumInputPorts=2
  Scope2 : Scope  NumInputPorts=2
  Scope3 : Scope  NumInputPorts=2
  Scope4 : Scope  Commented=on  NumInputPorts=2
  Scope5 : Scope  Commented=on  NumInputPorts=2
  Scope6 : Scope
  Scope7 : Scope
  Scope8 : Scope
  Sum1 : Sum  Commented=on  Inputs=+|-
  Sum2 : Sum  Inputs=+|-
  Sum3 : Sum  Commented=on  Inputs=+|-
  Sum4 : Sum  Inputs=+|-
  Sum6 : Sum  Commented=on  Inputs=+|-
  To Workspace : ToWorkspace  Commented=on  VariableName=rLoc2  SaveFormat=Timeseries  SampleTime=tSampData
  To Workspace1 : ToWorkspace  Commented=on  VariableName=rLoc_bar2  SaveFormat=Timeseries  SampleTime=tSampData
  To Workspace10 : ToWorkspace  Commented=on  VariableName=atkFlag42  SaveFormat=Timeseries  SampleTime=tSampData
  To Workspace2 : ToWorkspace  Commented=on  VariableName=r12  SaveFormat=Timeseries  SampleTime=tSampData
  To Workspace3 : ToWorkspace  Commented=on  VariableName=r_bar12  SaveFormat=Timeseries  SampleTime=tSampData
  To Workspace4 : ToWorkspace  Commented=on  VariableName=r_bar42  SaveFormat=Timeseries  SampleTime=tSampData
  To Workspace7 : ToWorkspace  Commented=on  VariableName=r42  SaveFormat=Timeseries  SampleTime=tSampData
  To Workspace8 : ToWorkspace  Commented=on  VariableName=atkFlagLoc2  SaveFormat=Timeseries  SampleTime=tSampData
  To Workspace9 : ToWorkspace  Commented=on  VariableName=atkFlag12  SaveFormat=Timeseries  SampleTime=tSampData
  tag scope: atkFlag12=global, atkFlag42=global, atkFlagLoc2=global, r12=global, r42=global, rLoc2=global
  wires:
  [secondary] -> Product2/2
  Sum2/1 -> Abs1/1
  Abs1/1 -> Product2/1
  [xhat2] -> Sum2/2
  Product2/1 -> [rLoc2]
  [y2] -> Sum2/1
  Sum6/1 -> Abs/1
  From2/1 -> Gain2/1
  Gain2/1 -> Scope4/2, Sum6/2
  From39/1 -> Scope4/1, Sum6/1
  Abs/1 -> Product/1
  Product/1 -> Goto2/1
  From1/1 -> Product/2
  Gain1/1 -> Scope5/2, Sum1/2
  From4/1 -> Gain1/1
  Product1/1 -> Goto1/1
  Sum1/1 -> Abs2/1
  From3/1 -> Product1/2
  Abs2/1 -> Product1/1
  From5/1 -> Scope5/1, Sum1/1
  Relational Operator1/1 -> Logical Operator1/1
  [rLoc_bar] -> Gain4/1
  Logical Operator1/1 -> To Workspace9/1, Scope7/1, [atkFlag12]
  [rLoc2] -> Relational Operator/1
  Relational Operator/1 -> Logical Operator/1
  [r_bar] -> Gain14/1
  Gain14/1 -> Relational Operator1/2
  Logical Operator/1 -> To Workspace8/1, Scope6/1, [atkFlagLoc2]
  [r12] -> Relational Operator1/1
  Relational Operator2/1 -> Logical Operator2/1
  Gain4/1 -> Relational Operator/2
  Gain15/1 -> Relational Operator2/2
  [r42] -> Relational Operator2/1
  [r_bar] -> Gain15/1
  Logical Operator2/1 -> To Workspace10/1, Scope8/1, [atkFlag42]
  [r_bar] -> Gain7/1
  [r_bar] -> Gain8/1
  [rLoc2] -> To Workspace/1, Scope2/1
  [r12] -> To Workspace2/1, Scope1/1
  Gain7/1 -> To Workspace3/1, Scope1/2
  Gain8/1 -> To Workspace4/1, Scope3/2
  Gain3/1 -> To Workspace1/1, Scope2/2
  [r42] -> To Workspace7/1, Scope3/1
  [rLoc_bar] -> Gain3/1
  From29/1 -> Product4/2
  From27/1 -> Sum3/2
  From28/1 -> Sum3/1
  Sum3/1 -> Abs4/1
  Product4/1 -> Gain9/1, Gain10/1
  Abs4/1 -> Product4/1
  Gain9/1 -> Goto7/1
  Gain10/1 -> Goto3/1
  Gain11/1 -> [r42]
  Gain12/1 -> [r12]
  Abs3/1 -> Product3/1
  Product3/1 -> Gain11/1, Gain12/1
  Sum4/1 -> Abs3/1
  [yComm2] -> Sum4/1
  [secondary] -> Product3/2
  [xbar2] -> Gain13/1
  Gain13/1 -> Sum4/2

== system simulation_w_switch_sln3/DGU2/Luenberger  Observer ==
  Gain1 : Gain  Gain=bigCyComm  Multiplication=Matrix(K*u) (u vector)
  Gain17 : Gain  Gain=[DGU(2).B , DGU(2).Li , DGU(2).M , Aij(1*n+1:2*n,:)]  Multiplication=Matrix(K*u) (u vector)
  Gain18 : Gain  Gain=DGU(2).A-DGU(2).Li*DGU(2).C  Multiplication=Matrix(K*u) (u vector)
  Integrator4 : Integrator  ExternalReset=rising  InitialConditionSource=external  InitialCondition=[0;0;0]
  Mux : Mux  Inputs=5
  Product4 : Product  Multiplication=Matrix(*)
  Sum10 : Sum  Inputs=++|
  tag scope: xhat2=global
  wires:
  Product4/1 -> [xhat2]
  [Il2] -> Mux/3
  [y2] -> Integrator4/3, Mux/2
  [Vref2] -> Mux/4
  Gain17/1 -> Sum10/2
  Gain18/1 -> Sum10/1
  [secondary] -> Integrator4/2, Product4/2
  Mux/1 -> Gain17/1
  Sum10/1 -> Integrator4/1
  Integrator4/1 -> Product4/1, Gain18/1
  [Vt2] -> Mux/1
  [yComm2] -> Gain1/1
  Gain1/1 -> Mux/5

== system simulation_w_switch_sln3/DGU2/Primary  Voltage  Controller ==
  Gain1 : Gain  Gain=DGU(2).K  Multiplication=Matrix(K*u) (u vector)
  tag scope: Vt2d=global
  wires:
  [y2] -> Gain1/1
  Gain1/1 -> [Vt2d]

== system simulation_w_switch_sln3/DGU2/Secondary  Consensus  Layer ==
  note: deltaV2
  Gain1 : Gain  Gain=repmat([0 0 0 0 1 0],1,6)  Multiplication=Matrix(K*u) (u vector)
  Gain13 : Gain  Gain=DGU(2).kI
  Gain7 : Gain  Gain=length(DGU(2).Ni)
  Integrator1 : Integrator  ExternalReset=rising
  Sum8 : Sum  Inputs=|+-
  Sum9 : Sum  Inputs=|++
  Switch1 : Switch  Criteria=u2 > Threshold  Threshold=0.1
  tag scope: Vref2=global
  wires:
  [It2] -> Gain7/1
  Gain7/1 -> Sum8/2
  Gain1/1 -> Sum8/1
  [yComm2] -> Gain1/1
  Integrator1/1 -> Sum9/1
  Sum9/1 -> Switch1/1
  Sum8/1 -> Gain13/1
  [secondary] -> Integrator1/2, Switch1/2
  Switch1/1 -> [Vref2]
  Gain13/1 -> Integrator1/1
  [Vref] -> Switch1/3, Sum9/2

== system simulation_w_switch_sln3/DGU2/Switching ==
  Divide : Product  Inputs=*/
  Logical Operator : Logic  Operator=NOT  AllPortsSameDT=off  OutDataTypeStr=boolean
  PWM Generator (DC-DC) : powerlib_meascontrol/Pulse & Signal Generators/PWM Generator (DC-DC)  Fsw=10000  Ts=0
  tag scope: SW_Buck_2=global, SW_Buck_2n=global, SW_Duty_2=global
  wires:
  [Vs2] -> Divide/2
  Logical Operator/1 -> [SW_Buck_2n]
  PWM Generator (DC-DC)/1 -> Logical Operator/1, [SW_Buck_2]
  Divide/1 -> [SW_Duty_2], PWM Generator (DC-DC)/1
  [Vt2d] -> Divide/1

== system simulation_w_switch_sln3/DGU2/UIO ==
  note: Single UIO for all neighbors of DGU 1 with Switched Inputs
  note: Calculated Switching Inputs
  note: 6x6 UIO for the states of DGUs with average dynamics
  Constant1 : Constant  Commented=on  Value=Vs
  Constant2 : Constant  Commented=on  Value=0.8132
  Divide : Product  Commented=on  Inputs=*/  Multiplication=Matrix(*)
  From5 : From  Commented=on  GotoTag=yComm2  TagVisibility=global
  From7 : From  Commented=on  GotoTag=yComm2  TagVisibility=global
  From8 : From  Commented=on  GotoTag=SW_yComm2  TagVisibility=global
  From9 : From  Commented=on  GotoTag=secondary  TagVisibility=global
  Gain15 : Gain  Gain=bH  Multiplication=Matrix(K*u) (u vector)
  Gain16 : Gain  Gain=inv(bC)-bH  Multiplication=Matrix(K*u) (u vector)
  Gain17 : Gain  Gain=bKhat  Multiplication=Matrix(K*u) (u vector)
  Gain18 : Gain  Gain=bF  Multiplication=Matrix(K*u) (u vector)
  Gain4 : Gain  Commented=on  Gain=K  Multiplication=Matrix(K*u) (u vector)
  Gain5 : Gain  Commented=on  Gain=[Khat T*B]  Multiplication=Matrix(K*u) (u vector)
  Gain6 : Gain  Commented=on  Gain=F  Multiplication=Matrix(K*u) (u vector)
  Gain7 : Gain  Commented=on  Gain=59.7999
  Gain8 : Gain  Commented=on  Gain=H  Multiplication=Matrix(K*u) (u vector)
  Gain9 : Gain  Commented=on  Gain=T  Multiplication=Matrix(K*u) (u vector)
  Goto : Goto  Commented=on  GotoTag=SW_yComm2  TagVisibility=global
  Goto3 : Goto  Commented=on  GotoTag=y_j2_hat  TagVisibility=global
  Goto4 : Goto  Commented=on  GotoTag=Duty_yComm2  TagVisibility=global
  Integrator1 : Integrator  Commented=on  ExternalReset=rising  InitialConditionSource=external
  Integrator4 : Integrator  ExternalReset=rising  InitialConditionSource=external  InitialCondition=[0;0;0]
  Mux3 : Mux  Commented=on  Inputs=2
  PWM Generator (DC-DC) : powerlib_meascontrol/Pulse & Signal Generators/PWM Generator (DC-DC)  Commented=on  Fsw=10000  Ts=0
  Product1 : Product  Commented=on  Multiplication=Matrix(*)
  Product4 : Product  Multiplication=Matrix(*)
  Sum10 : Sum  Inputs=++|
  Sum11 : Sum  Inputs=++|
  Sum2 : Sum  Commented=on  Inputs=++|
  Sum3 : Sum  Commented=on  Inputs=++|
  Sum4 : Sum  Commented=on  Inputs=|-+
  tag scope: xbar2=global
  wires:
  PWM Generator (DC-DC)/1 -> Goto/1
  Divide/1 -> Goto4/1, PWM Generator (DC-DC)/1
  Constant1/1 -> Divide/2
  Gain4/1 -> Divide/1
  From7/1 -> Gain4/1
  Constant2/1 -> Sum4/1
  From5/1 -> Gain8/1, Gain9/1, Mux3/1
  Sum3/1 -> Product1/1
  Gain5/1 -> Sum2/2
  Gain7/1 -> Sum4/2
  From8/1 -> Gain7/1
  Mux3/1 -> Gain5/1
  Gain8/1 -> Sum3/1
  Gain9/1 -> Integrator1/3
  From9/1 -> Integrator1/2, Product1/2
  Sum2/1 -> Integrator1/1
  Sum4/1 -> Mux3/2
  Integrator1/1 -> Sum3/2, Gain6/1
  Gain6/1 -> Sum2/1
  Product1/1 -> Goto3/1
  Sum11/1 -> Product4/1
  Gain18/1 -> Sum10/1
  Integrator4/1 -> Sum11/2, Gain18/1
  Gain17/1 -> Sum10/2
  Gain15/1 -> Sum11/1
  Product4/1 -> [xbar2]
  Sum10/1 -> Integrator4/1
  Gain16/1 -> Integrator4/3
  [yComm2] -> Gain16/1, Gain15/1, Gain17/1
  [secondary] -> Integrator4/2, Product4/2
